simulink model "ship_Berth"  (Simulink 10.3)
settings: Solver=ode23  StartTime=0.0  StopTime=1600  FixedStep=0.1  RelTol=1e-3  EnableMultiTasking=on
libraries: simulink x1
settings Model: Creator=Administrator  LastModifiedBy=1179956468
settings DataIOCC: LimitDataPoints=on
settings DebuggingCC: FcnCallInpInsideContextMsg=error
settings ConfigComp: CovSFcnEnable=off

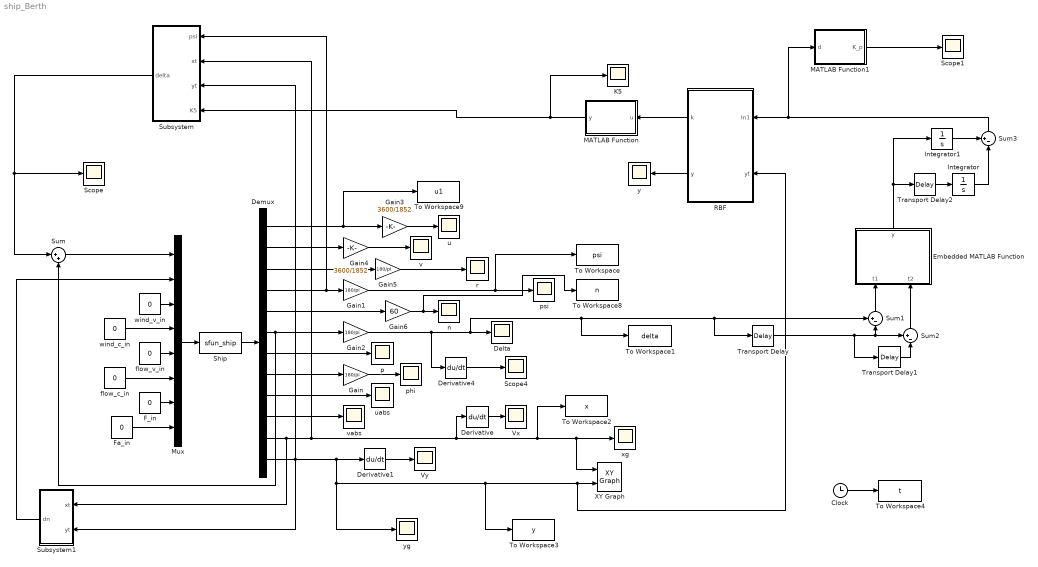
== system ship_Berth ==
  Clock : Clock
  Delta : Scope
  Demux : Demux  Outputs=12
  Derivative : Derivative
  Derivative1 : Derivative
  Derivative4 : Derivative
  Embedded MATLAB Function : MATLAB Function  TreatAsAtomicUnit=on
  F_in : Constant  Value=0
  Fa_in : Constant  Value=0
  Gain{,1..2,5} (4 alike) : Gain  Gain=180/pi
  Gain3 : Gain  Gain=3600/1852
  Gain4 : Gain  Gain=3600/1852
  Gain6 : Gain  Gain=60
  Integrator : Integrator
  Integrator1 : Integrator
  K5 : Scope
  MATLAB Function : MATLAB Function  TreatAsAtomicUnit=on
  MATLAB Function1 : MATLAB Function  TreatAsAtomicUnit=on
  Mux : Mux  Inputs=8
  RBF : Subsystem
  Scope : Scope
  Scope1 : Scope
  Scope4 : Scope
  Ship : S-Function  FunctionName=sfun_ship  SFunctionDeploymentMode=off  EnableBusSupport=off
  Subsystem : Subsystem
  Subsystem1 : Subsystem
  Sum : Sum  Inputs=|++
  Sum1 : Sum  Inputs=+-|
  Sum2 : Sum  Inputs=+-|
  Sum3 : Sum  Inputs=+-|
  To Workspace : ToWorkspace  VariableName=psi  SampleTime=-1
  To Workspace1 : ToWorkspace  VariableName=delta  SampleTime=-1
  To Workspace2 : ToWorkspace  VariableName=x  SampleTime=-1
  To Workspace3 : ToWorkspace  VariableName=y  SampleTime=-1
  To Workspace4 : ToWorkspace  VariableName=t  SampleTime=-1
  To Workspace8 : ToWorkspace  VariableName=n  SampleTime=-1
  To Workspace9 : ToWorkspace  VariableName=u1  SampleTime=-1
  Transport Delay : TransportDelay
  Transport Delay1 : TransportDelay
  Transport Delay2 : TransportDelay  DelayTime=50
  "Vx " : Scope
  Vy : Scope
  XY Graph : simulink/Sinks/XY Graph  xmin=-3000  xmax=3000  ymin=-3000  ymax=3000  st=-1
  flow_c_in : Constant  Value=0
  flow_v_in : Constant  Value=0
  n : Scope
  p : Scope
  phi : Scope
  psi : Scope
  r : Scope
  u : Scope
  uabs : Scope
  v : Scope
  vabs : Scope
  wind_c_in : Constant  Value=0
  wind_v_in : Constant  Value=0
  xg : Scope
  y : Scope
  yg : Scope
  wires:
  Ship/1 -> Demux/1
  Demux/1 -> Gain3/1, To Workspace9/1
  Demux/2 -> Gain4/1
  Demux/3 -> Gain5/1
  Demux/5 -> Gain6/1
  Demux/6 -> Gain2/1, Sum/2
  Demux/7 -> p/1
  Demux/8 -> Gain/1
  Gain1/1 -> psi/1, To Workspace/1
  Gain/1 -> phi/1
  Gain3/1 -> u/1
  Gain4/1 -> v/1
  Gain5/1 -> r/1
  Gain6/1 -> To Workspace8/1, n/1
  Demux/9 -> uabs/1
  Demux/10 -> vabs/1
  Demux/12 -> Derivative1/1, yg/1, To Workspace3/1, RBF/2(yt), XY Graph/2, Subsystem1/2(yt), Subsystem/3(yt)
  Demux/11 -> Subsystem/2(xt), Derivative/1, To Workspace2/1, XY Graph/1, xg/1, Subsystem1/1(xt)
  Derivative/1 -> "Vx "/1
  Derivative1/1 -> Vy/1
  wind_v_in/1 -> Mux/3
  wind_c_in/1 -> Mux/4
  flow_v_in/1 -> Mux/5
  F_in/1 -> Mux/7
  Fa_in/1 -> Mux/8
  Mux/1 -> Ship/1
  Derivative4/1 -> Scope4/1
  Demux/4 -> Gain1/1, Subsystem/1(psi)
  Subsystem1/1(dn) -> Mux/2
  Subsystem/1(delta) -> Sum/1, Scope/1
  Sum/1 -> Mux/1
  flow_c_in/1 -> Mux/6
  Clock/1 -> To Workspace4/1
  Gain2/1 -> Derivative4/1, Delta/1, Transport Delay/1, Sum1/1, To Workspace1/1
  Transport Delay/1 -> Sum1/2, Sum2/1, Transport Delay1/1
  Sum1/1 -> Embedded MATLAB Function/1(t1)
  Transport Delay1/1 -> Sum2/2
  Sum2/1 -> Embedded MATLAB Function/2(t2)
  Embedded MATLAB Function/1(y) -> Transport Delay2/1, Integrator1/1
  Transport Delay2/1 -> Integrator/1
  Integrator1/1 -> Sum3/1
  Integrator/1 -> Sum3/2
  Sum3/1 -> MATLAB Function1/1(d), RBF/1(In1)
  RBF/2(y) -> y/1
  RBF/1(k) -> MATLAB Function/1(u)
  MATLAB Function/1(y) -> K5/1, Subsystem/4(K5)
  MATLAB Function1/1(K_p) -> Scope1/1

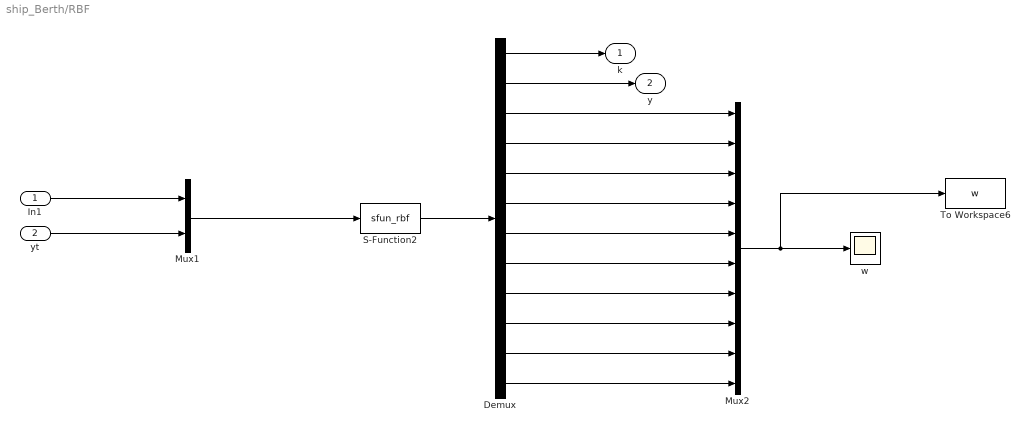
== system ship_Berth/RBF ==
  In1 : Inport
  yt : Inport  Port=2
  Demux : Demux  Outputs=12
  Mux1 : Mux  Inputs=2
  Mux2 : Mux  Inputs=10
  S-Function2 : S-Function  FunctionName=sfun_rbf  SFunctionDeploymentMode=off  EnableBusSupport=off
  To Workspace6 : ToWorkspace  VariableName=w  SampleTime=-1
  w : Scope
  k : Outport
  y : Outport  Port=2
  wires:
  In1/1 -> Mux1/1
  yt/1 -> Mux1/2
  Demux/1 -> k/1
  Demux/2 -> y/1
  Mux1/1 -> S-Function2/1
  Demux/3 -> Mux2/1
  Demux/4 -> Mux2/2
  Demux/5 -> Mux2/3
  Demux/6 -> Mux2/4
  Demux/7 -> Mux2/5
  Demux/8 -> Mux2/6
  Demux/9 -> Mux2/7
  Demux/10 -> Mux2/8
  Demux/11 -> Mux2/9
  Demux/12 -> Mux2/10
  Mux2/1 -> To Workspace6/1, w/1
  S-Function2/1 -> Demux/1

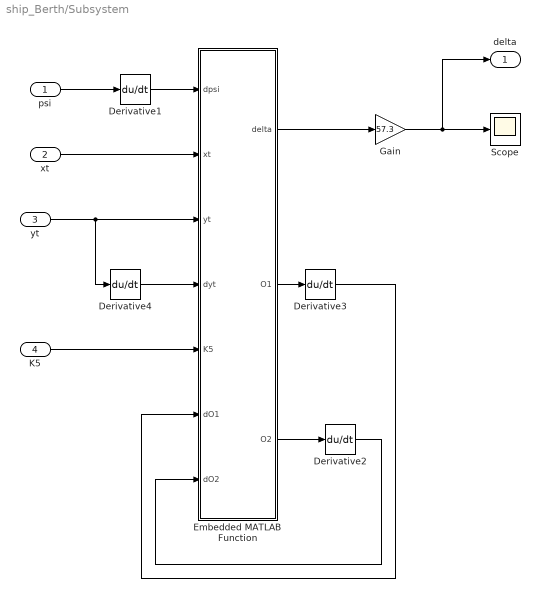
== system ship_Berth/Subsystem ==
  psi : Inport
  xt : Inport  Port=2
  yt : Inport  Port=3
  K5 : Inport  Port=4
  Derivative{1..4} (4 alike) : Derivative
  Embedded MATLAB Function : MATLAB Function  TreatAsAtomicUnit=on
  Gain : Gain  Gain=57.3
  Scope : Scope
  delta : Outport
  wires:
  Derivative2/1 -> Embedded MATLAB Function/7(dO2)
  psi/1 -> Derivative1/1
  xt/1 -> Embedded MATLAB Function/2(xt)
  yt/1 -> Derivative4/1, Embedded MATLAB Function/3(yt)
  Embedded MATLAB Function/1(delta) -> Gain/1
  Gain/1 -> delta/1, Scope/1
  Derivative4/1 -> Embedded MATLAB Function/4(dyt)
  Derivative1/1 -> Embedded MATLAB Function/1(dpsi)
  Embedded MATLAB Function/3(O2) -> Derivative2/1
  Embedded MATLAB Function/2(O1) -> Derivative3/1
  Derivative3/1 -> Embedded MATLAB Function/6(dO1)
  K5/1 -> Embedded MATLAB Function/5(K5)

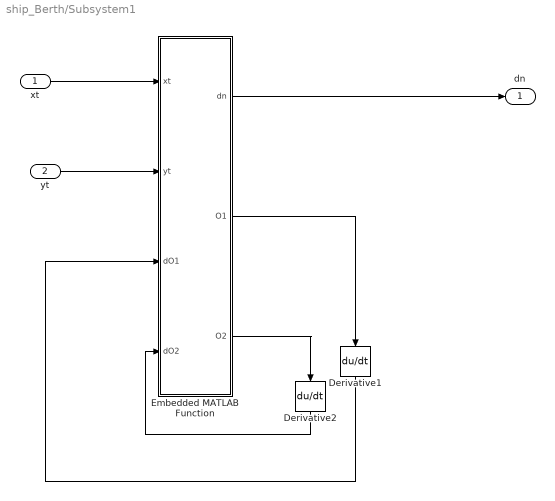
== system ship_Berth/Subsystem1 ==
  xt : Inport
  yt : Inport  Port=2
  Derivative1 : Derivative
  Derivative2 : Derivative
  Embedded MATLAB Function : MATLAB Function  TreatAsAtomicUnit=on
  dn : Outport
  wires:
  Embedded MATLAB Function/1(dn) -> dn/1
  xt/1 -> Embedded MATLAB Function/1(xt)
  Embedded MATLAB Function/2(O1) -> Derivative1/1
  Derivative1/1 -> Embedded MATLAB Function/3(dO1)
  yt/1 -> Embedded MATLAB Function/2(yt)
  Embedded MATLAB Function/3(O2) -> Derivative2/1
  Derivative2/1 -> Embedded MATLAB Function/4(dO2)

== matlab function Subsystem1/Embedded MATLAB Function ==
  data: dn output double; xt input double; yt input double; dO1 input double; O1 output double; O2 output double; dO2 input double
function [dn,O1,O2]=fcn(xt,yt,dO1,dO2)
K1=10;K2=1;K3=0.01;K4=50;K5=0.0018;K6=0;Tm=4;
%K11=3500;K12=3;K13=0.01;K14=0.0000005;K15=0.00006;K16=0;Tm=4;

O1=xt-yt;
O2=K1*tanh(K2*O1)+dO1;
O3=K3*tanh(K4*O2)+dO2;
dn=-K5*O3-K6*tanh(O3);
%function q=sgn(a)
 % if (a>0)
  %    q=1;
  %else
   %   q=-1;
  %end
%nr=n+Tm*dn;

== matlab function Subsystem/Embedded MATLAB Function ==
  data: delta output double; O1 output double; dpsi input double; xt input double; yt input double; dyt input double; K5 input double; dO1 input double; O2 output double; dO2 input double
function [delta,O1,O2] = fcn(dpsi,xt,yt,dyt,K5,dO1,dO2)

%K0=0.2;K1=0.005;K2=0.0004;K3=0.0000005;K4=3.4;K5=130;Te=2.5;
K1=2;K2=0.01;K3=3;K4=0.1;K6=0;Te=2.5;
% K5=2;

O1=K1*f(K2*yt)+dyt;
O2=dpsi+K3*f(O1);
O3=K4*f(O2)+dO2;
%delta=-K5*O3-K6*f(O3);%用舵机模型总是出错
delta=-Te*K5*O3;
 function mean=f(a)
  mean=tanh(a);
%  function mean=f(a)
%  if(a<0.1&&a>-0.1)
%      mean=a;
%  else
%      mean=coth(a)-1/a;
%  end

== matlab function Embedded MATLAB Function ==
  data: t1 input double; y output double; t2 input double
function y = fcn(t1,t2)
%#eml
if(t1*t2>0)
  p=0;
else
    p=1;
end
y = p*t1;

== matlab function MATLAB Function ==
  data: u input double; y output double
function y = fcn(u)
%#codegen
% if(u>5||u<1)
% y = u;
% else
%     y=2;
% end
y=2;

== matlab function MATLAB Function1 ==
  data: d input double; K_p output double

function K_p  = fcn(d)
%#codegen
w = 0.01*(d-0.5)/0.5;%0.6;      % 惯性因子 
c1 = 2;       % 加速常数
c2 = 2;       % 加速常数

Dim = 1;            % 维数
SwarmSize = 100;    % 粒子群规模
%ObjFun = @PSO_PID;  % 待优化函数句柄

MaxIter = 100;      % 最大迭代次数  
MinFit = 0.1;       % 最小适应值 

Vmax = 1;
Vmin = -1;
Ub = 30;
Lb = 0;

% 粒子群初始化
    Range = ones(SwarmSize,1)*(Ub-Lb);
    Swarm = rand(SwarmSize,Dim).*Range + ones(SwarmSize,1)*Lb ;     % 初始化粒子群      
    VStep = rand(SwarmSize,Dim)*(Vmax-Vmin) + Vmin     ;            % 初始化速度        
    fSwarm = zeros(SwarmSize,1);
for i=1:SwarmSize
    fSwarm(i,:) = sum(Swarm(i,:) ^ 2 - 10 * cos( 2 * pi * Swarm(i,:)) + 10 );%feval(ObjFun,Swarm(i,:));                         % 粒子群的适应值%%%%%%%%%%%%%%%%%%%%%%%%%%%%%%%%%%%%%%%%%%%%%%%%%%%%%%%%%
end

%% 个体极值和群体极值
[bestf, bestindex]=min(fSwarm);
zbest=Swarm(bestindex,:);   % 全局最佳
gbest=Swarm;                % 个体最佳
fgbest=fSwarm;              % 个体最佳适应值
fzbest=bestf;               % 全局最佳适应值

%% 迭代寻优
iter = 0;
y_fitness = zeros(1,MaxIter);   % 预先产生4个空矩阵
K_p = zeros(1,MaxIter);         

while( (iter < MaxIter) && (fzbest > MinFit) )
    for j=1:SwarmSize
        % 速度更新
        VStep(j,:) = w*VStep(j,:) + c1*rand*(gbest(j,:) - Swarm(j,:)) + c2*rand*(zbest - Swarm(j,:));
        if VStep(j,:)>Vmax, VStep(j,:)=Vmax; end
        if VStep(j,:)<Vmin, VStep(j,:)=Vmin; end
        % 位置更新
        Swarm(j,:)=Swarm(j,:)+VStep(j,:);
        for k=1:Dim
            if Swarm(j,k)>Ub(k), Swarm(j,k)=Ub(k); end
            if Swarm(j,k)<Lb(k), Swarm(j,k)=Lb(k); end
        end
        % 适应值
        fSwarm(j,:) =sum(Swarm(i,:) ^ 2 - 10 * cos( 2 * pi * Swarm(i,:)) + 10 ); %feval(ObjFun,Swarm(j,:));
        % 个体最优更新     
        if fSwarm(j) < fgbest(j)
            gbest(j,:) = Swarm(j,:);
            fgbest(j) = fSwarm(j);
        end
        % 群体最优更新
        if fSwarm(j) < fzbest
            zbest = Swarm(j,:);
            fzbest = fSwarm(j);
        end
    end 
    iter = iter+1;                      % 迭代次数更新
    y_fitness(1,iter) = fzbest;         % 为绘图做准备
    K_p(1,iter) =  fzbest;%*[0 0 0 0 0 0 0 0 0 0 0 0 0 0 0 0 0 0 0 0 0 0 0 0 0 0 0 0 0 0 0 0 0 0 0 0 0 0 0 0 0 0 0 0 0 0 0 0 0 0 0 0 0 0 0 0 0 0 0 0 0 0 0 0 0 0 0 0 0 0 0 0 0 0 0 0 0 0 0 0 0 0 0 0 0 0 0 0 0 0 0 0 0 0 0 0 0 0 0 1]'; %zbest(1);

end
